simulink model "ComplexPhaseDetectorSwap"  (R2016a)
settings: Solver=VariableStepAuto  StartTime=0.0  StopTime=.05  RelTol=1e-6
PreLoadFcn:
  | Bits = 4
  | Ts=2*3/280e6
  | dBRange=11
  | maxNumErrs=500
  | maxNumBits=1e6
  | AM_Gain=AM_GainDiff;
  | AGC_Gain=AGC_GainCalc;
  | load('IIR_Coeffs.mat');
InitFcn:
  | Br= 1/(10*Ts)
  | FreqOffset=00
  | Mode=2
  | BitsPer=[2,2,1,1]
  | EbNo=50
  | N=6
undefined symbols (not defined in the file or in its folder): designMultirateFIR, DiscIntNeverNeededParam
libraries: xbsIndex_r4 x792, commfilt2 x12, commsink2 x6, dspsigops x4, commrfcorlib x2, commchan3 x2, dspfdesign x2, dspstat3 x2, dspmlti4 x1, commdigbbndpm3 x1, commrandsrc3 x1
(part 1 of 10)
settings Model: Creator=frank.ziegler  LastModifiedBy=frank
settings DebuggingCC: ConsistencyChecking=warning  ArrayBoundsChecking=error  UniqueDataStoreMsg=error

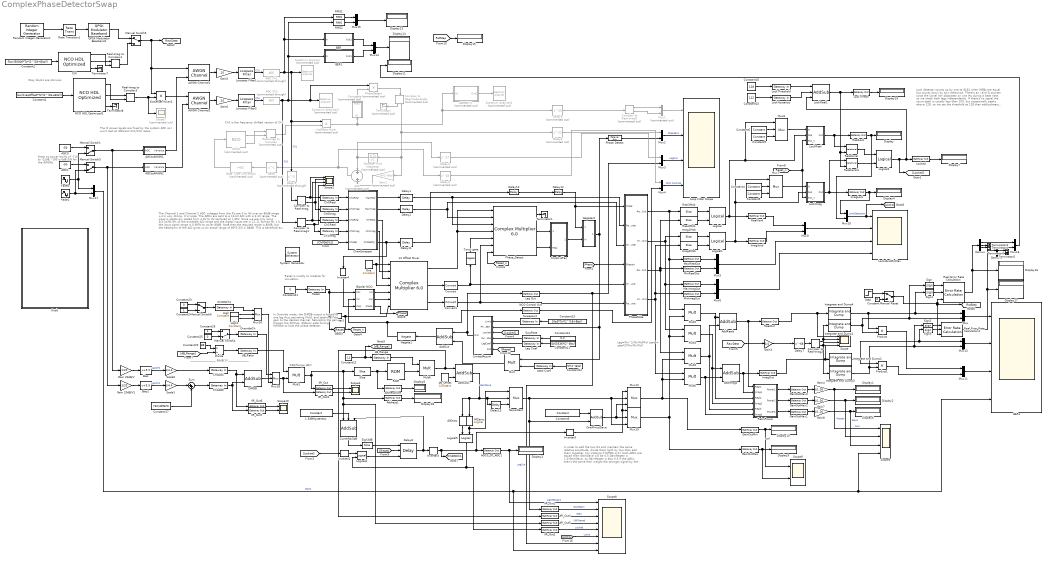
== system ComplexPhaseDetectorSwap ==
  note: Lag=Wn^2/(Kv*Kd*Fs)
      | Lead = zeta*2*Wn/(Kv*Kd)
  note: Lock detector counts up by one to 8191 when MSBs are equal but counts down by two otherwise. There's an I and Q counter since the signal can disappear on one leg during a beat note, so we check both legs independently. If there's no signal the count peak is usually less than 100, but occasionally peaks above 128, so we set the threshold at 128 then add/subtract 112 of hysterisis such that both signals have to drop below 16 to loose lock, then either rise above 240. This gives a strong confidence to the lock and allows the 8192 a long time (76uS) to count down to 256 during a fade.
      | Note, the higher the beat note in the IF, the more false negative at high noise levels. At 800Hz I've seen an error every 10 seconds or so.
  note: Reset is mostly to initialize for simulation
  note: Enter as power levels of -110 to -22dB.
      | -100 is 0dB S/N for the AWGNs
  note: The IF power levels are fixed by the system AGC so I won't test at different Ch1/Ch2 ratios.
  note: Ch2 is the frequency shifted version of Ch1.
  note: The Channel 1 and Channel 2 AGC voltages from the IFs are 0 to 4V over an 80dB range. +4 is very strong, 0 is noise. The AGCs are sent to a 12-bit A/D with a 3.3V range. The input is resistively scaled from 4.0V to 3V centered at 1.65V. Since we are only using 3/3.3=90.9% of the available A/D range and the digital inputs are in 12.11 format for 1.0, the input signal range is 0.909V to cover 80dB.
      | Note that the required range is 80dB, but the headroom of the A/D gives us an actual range of 80*3.3/3 = 88dB. This is beneficial as shown below.
      | We take the difference in AGC voltage between the two channels to define the weighting system based on the stronger signal. If we take the differential and multiply by 8 with saturation this effectively gives us a ± 11dB differential maximum. We can use this to limit the range the combiner attempts to work over since combining is only useful over a 10dB range. The nature of the saturation forces a "Best Source Select" function automatically. We take the sign to define the larger channel. The value addresses a look up table that does the log to linear conversion over a 16384-bit resolution. The Log2Lin transposes the log nature of the AGC to a linear ratio of the two signals. If the two AGCs are the same, the differential is zero and the weights are set to 50-50 for optimal combining. As the difference approaches +1.0, the largest signal gets a weight of 100%.and the other is shut off with a weight of 0%.
  note: In order to add the two IFs and maintain the same relative amplitude, divide them both by two then add them together.
      | For instance if DiffDb is 0 ( both AGCs are equal) then GainSlave will be 0.5.GainMaster = 1.0-GainSlave, so GainMaster is also 0.5
      | If the AGCs aren't the same then weight the stronger signal by the differential.
      | If  GainSlave saturates, ignore the lock and pick the larger signal immediately
  note: In Override mode, the DiffDB output is forced to one leg thus saturating Mult1 and setting all the gain to the desired channel. Saturating the gain triggers the AllOnes, AllZeros gate forcing HardSel to hold the phase detector.
  note: ±88/Range dB/V
  note: ___________________ 88dB/1V _______________
  note: Grey blocks are stimulus
  " System Generator" : xbsIndex_r4/ System Generator  Tag=genX  xilinxfamily=kintex7  part=xc7k325t  speed=-2  package=fbg676  synthesis_tool=Vivado  clock_wrapper=Clock Enables  directory=./netlist  proj_type=Vivado  Synth_file=Vivado Synthesis Defaults  Impl_file=Vivado Implementation Defaults  testbench=off  simulink_period=Ts  sysclk_period=2*3000/280  dcm_input_clock_period=10  incr_netlist=off  trim_vbits=Everywhere in SubSystem  dbl_ovrd=According to Block Masks  core_generation=According to Block Masks  run_coregen=off  deprecated_control=off  eval_field=0  block_type=sysgen
  1.5dBHysteresis : xbsIndex_r4/Constant  const=1.5/11  gui_display_data_type=Fixed-point  arith_type=Signed (2's comp)  n_bits=18  bin_pt=17  preci_type=Single  exp_width=8  frac_width=24  explicit_period=on  period=Ts  equ=P=C  opselect=C  inp2=PCIN>>17  opr=+  inp1=P  carry=CIN  dbl_ovrd=off  block_type=constant
  AD9957-2 : Subsystem  Commented=on
  AGC Ch1 : commrfcorlib/AGC  Commented=through  LegacyMode=off  DetectorMethod=Rectifier  LoopMethod=Linear  UpdatePeriod=100  StepSize=0.1  AdaptationStepSize=0.001  DesiredOutputPower=.05  AveragingLength=100  MaximumGain=30  MaxPowerGain=6  GainOutputPort=off  InputPowerOutputPort=off  SimulateUsing=Interpreted execution
  AGC Ch2 : commrfcorlib/AGC  Commented=through  LegacyMode=off  DetectorMethod=Rectifier  LoopMethod=Linear  UpdatePeriod=100  StepSize=0.1  AdaptationStepSize=0.001  DesiredOutputPower=.05  AveragingLength=100  MaximumGain=30  MaxPowerGain=6  GainOutputPort=off  InputPowerOutputPort=off  SimulateUsing=Interpreted execution
  AGC0 : Constant  Value=-50  OutDataTypeStr=double
  AGC0_GT_AGC1 : xbsIndex_r4/Gateway Out  inherit_from_input=off  hdl_port=on  rows=1  columns=1  UseAsDAC=off  DACChannel='1'  interface=None  automatic_assignment=on  address_offset=hex2dec('00')  intf_name=''  intf_description=''  timing_constraint=None  locs_specified=off  LOCs={}  io_standard={}  block_type=gatewayout
  AGC1 : Constant  Value=-50  OutDataTypeStr=double
  AGCtoAWGN1 : Subsystem
  AGCtoAWGN2 : Subsystem
  AWGN Channel1 : commchan3/AWGN Channel  InputProcessing=Columns as channels (frame based)  seed=67  noiseMode=Variance from port  EbNodB=4  EsNodB=10  SNRdB=10  bitsPerSym=BitsPer(Mode)  Ps=0.707  Tsym=1/Br  variance=1
  AWGN Channel2 : commchan3/AWGN Channel  InputProcessing=Columns as channels (frame based)  seed=70  noiseMode=Variance from port  EbNodB=6  EsNodB=10  SNRdB=10  bitsPerSym=BitsPer(Mode)  Ps=0.707  Tsym=1/Br  variance=1
  Add : Sum  Commented=on  OutDataTypeStr=Inherit: Same as first input
  AddImags : xbsIndex_r4/AddSub  mode=Addition  use_carryin=off  use_carryout=off  en=off  latency=1  precision=User Defined  arith_type="Signed  (2's comp)"  n_bits=18  bin_pt=17  quantization="Round  (unbiased: +/- Inf)"  overflow=Saturate  use_behavioral_HDL=off  hw_selection=Fabric  pipelined=off  dbl_ovrd=off  block_type=addsub
  AddReals : xbsIndex_r4/AddSub  mode=Addition  use_carryin=off  use_carryout=off  en=off  latency=1  precision=User Defined  arith_type="Signed  (2's comp)"  n_bits=18  bin_pt=17  quantization="Round  (unbiased: +/- Inf)"  overflow=Saturate  use_behavioral_HDL=off  hw_selection=Fabric  pipelined=off  dbl_ovrd=off  block_type=addsub
  AddSub : xbsIndex_r4/AddSub  mode=Addition  use_carryin=off  use_carryout=off  en=off  latency=1  precision=User Defined  arith_type="Signed  (2's comp)"  n_bits=18+Bits  bin_pt=0  quantization=Truncate  overflow=Wrap  use_behavioral_HDL=off  hw_selection=Fabric  pipelined=off  dbl_ovrd=off  block_type=addsub
  AddSub1 : xbsIndex_r4/AddSub  mode=Addition  use_carryin=off  use_carryout=off  en=off  latency=1  precision=User Defined  arith_type=Unsigned  n_bits=18  bin_pt=18  quantization=Truncate  overflow=Saturate  use_behavioral_HDL=off  hw_selection=Fabric  pipelined=off  dbl_ovrd=off  block_type=addsub
  Address1 : xbsIndex_r4/Gateway Out  inherit_from_input=off  hdl_port=off  rows=1  columns=1  UseAsDAC=off  DACChannel='1'  interface=None  automatic_assignment=on  address_offset=hex2dec('00')  intf_name=''  intf_description=''  timing_constraint=None  locs_specified=off  LOCs={}  io_standard={}  block_type=gatewayout
  AddressSlice : xbsIndex_r4/Gateway Out  inherit_from_input=off  hdl_port=off  rows=1  columns=1  UseAsDAC=off  DACChannel='1'  interface=None  automatic_assignment=on  address_offset=hex2dec('00')  intf_name=''  intf_description=''  timing_constraint=None  locs_specified=off  LOCs={}  io_standard={}  block_type=gatewayout
  AllOnes : xbsIndex_r4/Logical  logical_function=AND  inputs=1  en=off  latency=0  precision=Full  arith_type=Unsigned  n_bits=16  bin_pt=0  align_bp=on  dbl_ovrd=off  block_type=logical
  AllZeros : xbsIndex_r4/Logical  logical_function=NOR  inputs=1  en=off  latency=0  precision=Full  arith_type=Unsigned  n_bits=16  bin_pt=0  align_bp=on  dbl_ovrd=off  block_type=logical
  BER : Subsystem
  BER1 : Subsystem
  BERs : Scope  NumInputPorts=4
  Bias : Bias  Bias=5.5
  Bias1 : Bias  Bias=5.5
  Bipolar NCO : Subsystem
  CW : dspsigops/NCO HDL Optimized  PhaseIncrementSource=Input port  PhaseIncrement=100  PhaseOffsetSource=Property  PhaseOffset=0  DitherSource=Property  NumDitherBits=4  PhaseQuantization=on  NumQuantizerAccumulatorBits=12  LUTCompress=off  ResetAction=off  ValidInputPort=off  Waveform=Sine and cosine  PhasePort=off  AccumulatorWL=18+Bits  OutputDataType=double  OutputWL=16  OutputFL=14  SimulateUsing=Code generation
  Ch0AGC : xbsIndex_r4/Gateway In  gui_display_data_type=Fixed-point  arith_type=Unsigned  n_bits=13  bin_pt=12  preci_type=Single  exp_width=8  frac_width=24  rows=1  columns=1  quantization="Round  (unbiased: +/- Inf)"  overflow=Saturate  period=Ts  UseAsADC=off  ADCChannel='1'  interface=None  automatic_assignment=on  address_offset=hex2dec('00')  intf_name=''  intf_description=''  default_value=0  timing_constraint=None  locs_specified=off  LOCs={}  io_standard={}  inherit_from_input=off  hdl_port=on  dbl_ovrd=off  block_type=gatewayin
  Ch0GtCh1 : xbsIndex_r4/Gateway In  gui_display_data_type=Boolean  arith_type=Boolean  n_bits=18  bin_pt=9  preci_type=Single  exp_width=8  frac_width=24  rows=1  columns=1  quantization="Round  (unbiased: +/- Inf)"  overflow=Wrap  period=Ts  UseAsADC=off  ADCChannel='1'  interface=None  automatic_assignment=on  address_offset=hex2dec('00')  intf_name='axi4'  intf_description='Lead Coefficient'  default_value=10  timing_constraint=None  locs_specified=off  LOCs={}  io_standard={}  inherit_from_input=off  hdl_port=on  dbl_ovrd=off  block_type=gatewayin
  Ch0Imag : xbsIndex_r4/Gateway In  gui_display_data_type=Fixed-point  arith_type="Signed  (2's comp)"  n_bits=18  bin_pt=17  preci_type=Single  exp_width=8  frac_width=24  rows=1  columns=1  quantization="Round  (unbiased: +/- Inf)"  overflow=Saturate  period=Ts  UseAsADC=off  ADCChannel='1'  interface=None  automatic_assignment=on  address_offset=hex2dec('00')  intf_name=''  intf_description=''  default_value=0  timing_constraint=None  locs_specified=off  LOCs={}  io_standard={}  inherit_from_input=off  hdl_port=on  dbl_ovrd=off  block_type=gatewayin
  Ch0Real : xbsIndex_r4/Gateway In  gui_display_data_type=Fixed-point  arith_type="Signed  (2's comp)"  n_bits=18  bin_pt=17  preci_type=Single  exp_width=8  frac_width=24  rows=1  columns=1  quantization="Round  (unbiased: +/- Inf)"  overflow=Saturate  period=Ts  UseAsADC=off  ADCChannel='1'  interface=None  automatic_assignment=on  address_offset=hex2dec('00')  intf_name=''  intf_description=''  default_value=0  timing_constraint=None  locs_specified=off  LOCs={}  io_standard={}  inherit_from_input=off  hdl_port=on  dbl_ovrd=off  block_type=gatewayin
  Ch1AGC : xbsIndex_r4/Gateway In  gui_display_data_type=Fixed-point  arith_type=Unsigned  n_bits=13  bin_pt=12  preci_type=Single  exp_width=8  frac_width=24  rows=1  columns=1  quantization="Round  (unbiased: +/- Inf)"  overflow=Saturate  period=Ts  UseAsADC=off  ADCChannel='1'  interface=None  automatic_assignment=on  address_offset=hex2dec('00')  intf_name=''  intf_description=''  default_value=0  timing_constraint=None  locs_specified=off  LOCs={}  io_standard={}  inherit_from_input=off  hdl_port=on  dbl_ovrd=off  block_type=gatewayin
  Ch1Imag : xbsIndex_r4/Gateway In  gui_display_data_type=Fixed-point  arith_type="Signed  (2's comp)"  n_bits=18  bin_pt=17  preci_type=Single  exp_width=8  frac_width=24  rows=1  columns=1  quantization="Round  (unbiased: +/- Inf)"  overflow=Saturate  period=Ts  UseAsADC=off  ADCChannel='1'  interface=None  automatic_assignment=on  address_offset=hex2dec('00')  intf_name=''  intf_description=''  default_value=0  timing_constraint=None  locs_specified=off  LOCs={}  io_standard={}  inherit_from_input=off  hdl_port=on  dbl_ovrd=off  block_type=gatewayin
  Ch1Real : xbsIndex_r4/Gateway In  gui_display_data_type=Fixed-point  arith_type="Signed  (2's comp)"  n_bits=18  bin_pt=17  preci_type=Single  exp_width=8  frac_width=24  rows=1  columns=1  quantization="Round  (unbiased: +/- Inf)"  overflow=Saturate  period=Ts  UseAsADC=off  ADCChannel='1'  interface=None  automatic_assignment=on  address_offset=hex2dec('00')  intf_name=''  intf_description=''  default_value=0  timing_constraint=None  locs_specified=off  LOCs={}  io_standard={}  inherit_from_input=off  hdl_port=on  dbl_ovrd=off  block_type=gatewayin
  ChanSwapper : Subsystem
  Complex to Magnitude-Angle : ComplexToMagnitudeAngle  Commented=on
  Complex to Real-Imag : ComplexToRealImag
  Complex to Real-Imag1 : ComplexToRealImag
  Complex to Real-Imag2 : ComplexToRealImag
  Complex to Real-Imag5 : ComplexToRealImag  Commented=on
  Conju gate : xbsIndex_r4/Negate  precision=User Defined  arith_type="Signed  (2's comp)"  n_bits=18  bin_pt=17  quantization=Truncate  overflow=Saturate  en=off  latency=0  dbl_ovrd=off  block_type=negate
  Conjugate : Subsystem  Commented=on
  Constant : Constant  Value=0
  Constant1 : Constant  Value=floor(FreqOffset*Ts*(2^(18+Bits)))  OutDataTypeStr=int32  SampleTime=Ts
  Constant10 : Constant  Value=128
  Constant11 : Constant  Value=50/65536*(2^Bits)  OutDataTypeStr=double
  Constant12 : Constant  Value=5*(2^Bits)  OutDataTypeStr=double
  Constant13 : Constant  Value=10e3*Ts*(2^(18+Bits))  OutDataTypeStr=double
  Constant14 : Constant  Value=0.2  OutDataTypeStr=double
  Constant15 : Constant  Value=112
  Constant17 : Constant  Value=732/4096*0
  Constant2 : Constant  Value=floor(50000*Ts*(2^(18+Bits)))  OutDataTypeStr=int32  SampleTime=Ts
  Constant20 : Constant  Value=88  OutDataTypeStr=double
  Constant21 : Constant  Value=0  OutDataTypeStr=double
  Constant22 : Constant  Value=11  OutDataTypeStr=double
  Constant23 : Constant  Value=0  OutDataTypeStr=double
  Constant24 : Constant  OutDataTypeStr=double
  Constant25 : Constant  Value=0  OutDataTypeStr=double
  Constant26 : Constant  OutDataTypeStr=double
  Constant3 : xbsIndex_r4/Constant  const=1.0  gui_display_data_type=Fixed-point  arith_type=Unsigned  n_bits=18  bin_pt=18  preci_type=Single  exp_width=8  frac_width=24  explicit_period=on  period=Ts  equ=P=C  opselect=C  inp2=PCIN>>17  opr=+  inp1=P  carry=CIN  dbl_ovrd=off  block_type=constant
  Constant4 : xbsIndex_r4/Constant  const=1  gui_display_data_type=Fixed-point  arith_type=Unsigned  n_bits=8  bin_pt=0  preci_type=Single  exp_width=8  frac_width=24  explicit_period=off  period=1  equ=P=C  opselect=C  inp2=PCIN>>17  opr=+  inp1=P  carry=CIN  dbl_ovrd=off  block_type=constant
  Constant5 : xbsIndex_r4/Constant  const=2  gui_display_data_type=Fixed-point  arith_type=Unsigned  n_bits=8  bin_pt=0  preci_type=Single  exp_width=8  frac_width=24  explicit_period=off  period=1  equ=P=C  opselect=C  inp2=PCIN>>17  opr=+  inp1=P  carry=CIN  dbl_ovrd=off  block_type=constant
  Constant6 : xbsIndex_r4/Constant  const=1  gui_display_data_type=Fixed-point  arith_type=Unsigned  n_bits=8  bin_pt=0  preci_type=Single  exp_width=8  frac_width=24  explicit_period=off  period=1  equ=P=C  opselect=C  inp2=PCIN>>17  opr=+  inp1=P  carry=CIN  dbl_ovrd=off  block_type=constant
  Constant9 : xbsIndex_r4/Constant  const=2  gui_display_data_type=Fixed-point  arith_type=Unsigned  n_bits=8  bin_pt=0  preci_type=Single  exp_width=8  frac_width=24  explicit_period=off  period=1  equ=P=C  opselect=C  inp2=PCIN>>17  opr=+  inp1=P  carry=CIN  dbl_ovrd=off  block_type=constant
  Convert : xbsIndex_r4/Convert  gui_display_data_type=Fixed-point  arith_type="Signed  (2's comp)"  n_bits=18  bin_pt=17  float_type=Single  exp_bits=8  fraction_bits=24  quantization=Truncate  overflow=Saturate  en=off  latency=1  pipeline=off  dbl_ovrd=off  block_type=convert
  Convert1 : xbsIndex_r4/Convert  gui_display_data_type=Fixed-point  arith_type="Signed  (2's comp)"  n_bits=18  bin_pt=17  float_type=Single  exp_bits=8  fraction_bits=24  quantization=Truncate  overflow=Saturate  en=off  latency=1  pipeline=off  dbl_ovrd=off  block_type=convert
  Cordic ATan : Subsystem
  Current±3dB : xbsIndex_r4/AddSub  mode=Addition or Subtraction  use_carryin=off  use_carryout=off  en=off  latency=0  precision=User Defined  arith_type="Signed  (2's comp)"  n_bits=12  bin_pt=11  quantization=Truncate  overflow=Saturate  use_behavioral_HDL=off  hw_selection=Fabric  pipelined=off  dbl_ovrd=off  block_type=addsub
  Data Type Conversion : DataTypeConversion  Commented=on  OutDataTypeStr=int32  SaturateOnIntegerOverflow=on
  Delay : Delay  Commented=on  DelayLength=1
  Delay1 : xbsIndex_r4/Delay  rst=off  infoeditControl=Selection of Reset will increase slice count due to use of real FFs and instead of SRLs  en=off  latency=4  reg_retiming=off  dbl_ovrd=off  block_type=delay
  Delay10 : xbsIndex_r4/Delay  rst=off  infoeditControl=Selection of Reset will increase slice count due to use of real FFs and instead of SRLs  en=off  latency=3  reg_retiming=off  dbl_ovrd=off  block_type=delay
  Delay11 : xbsIndex_r4/Delay  rst=off  infoeditControl=Selection of Reset will increase slice count due to use of real FFs and instead of SRLs  en=off  latency=4  reg_retiming=off  dbl_ovrd=off  block_type=delay
  Delay12 : xbsIndex_r4/Delay  rst=off  infoeditControl=Selection of Reset will increase slice count due to use of real FFs and instead of SRLs  en=off  latency=17  reg_retiming=off  dbl_ovrd=off  block_type=delay
  Delay13 : xbsIndex_r4/Delay  rst=off  infoeditControl=Selection of Reset will increase slice count due to use of real FFs and instead of SRLs  en=off  latency=1  reg_retiming=off  dbl_ovrd=off  block_type=delay
  Delay2 : xbsIndex_r4/Delay  rst=off  infoeditControl=Selection of Reset will increase slice count due to use of real FFs and instead of SRLs  en=off  latency=4  reg_retiming=off  dbl_ovrd=off  block_type=delay
  Delay3 : Delay  Commented=on  DelayLength=27
  Delay4 : Delay  Commented=on  DelayLength=28
  Delay5 : Delay  Commented=on  DelayLength=23
  Delay6 : Delay  Commented=on  DelayLength=23
  Delay7 : Delay  DelayLength=68
  Delay8 : xbsIndex_r4/Delay  rst=on  infoeditControl=Selection of Reset will increase slice count due to use of real FFs and instead of SRLs  en=on  latency=1  reg_retiming=off  dbl_ovrd=off  block_type=delay
  Delay9 : Delay  Commented=through  DelayLength=3
  Demux : Demux  Outputs=3
  Demux1 : Demux  Outputs=3
  DiffDB : xbsIndex_r4/AddSub  mode=Subtraction  use_carryin=off  use_carryout=off  en=off  latency=1  precision=Full  arith_type="Signed  (2's comp)"  n_bits=13  bin_pt=12  quantization=Truncate  overflow=Saturate  use_behavioral_HDL=off  hw_selection=Fabric  pipelined=off  dbl_ovrd=off  block_type=addsub
  Discrete-Time Integrator : DiscreteIntegrator  Commented=on  gainval=(2^Bits)*50/65536/Ts  InitialConditionSetting=State (most efficient)  SampleTime=Ts  ICPrevOutput=DiscIntNeverNeededParam  ICPrevScaledInput=DiscIntNeverNeededParam
  Display{,1..4,6..11,13..19} (18 alike) : Display
      Display11 settings: Format=short_e
      Display14 settings: Format=short_e
  Divide : Product  Inputs=*/
  ExtOffset Mixer1 : Product
  Fade0 : Sin  Amplitude=10  Bias=-90  Frequency=5000*pi()  SampleTime=Ts
  Fade1 : Sin  Amplitude=10  Bias=-90  Frequency=5000*pi()  Phase=pi()  SampleTime=Ts
  Gain 20dB/V : Gain  Gain=1/20
  Gain 20dB/V1 : Gain  Gain=1/20
  Gain1 : Gain  Commented=on  Gain=5*(2^Bits)
  Gain3 : Gain  Gain=1/4
  Gain4 : Gain  Gain=1/1.26
  Gain5 : Gain  Gain=.25
  Gain6 : Gain  Gain=.25
  Gain7 : Gain  Gain=1/1.26
  Gain8 : Gain  Gain=1/1.26
  GainOutMax : xbsIndex_r4/Gateway Out  inherit_from_input=off  hdl_port=on  rows=1  columns=1  UseAsDAC=off  DACChannel='1'  interface=None  automatic_assignment=on  address_offset=hex2dec('00')  intf_name=''  intf_description=''  timing_constraint=None  locs_specified=off  LOCs={}  io_standard={}  block_type=gatewayout
  GainOutMax1 : xbsIndex_r4/Gateway Out  inherit_from_input=off  hdl_port=off  rows=1  columns=1  UseAsDAC=off  DACChannel='1'  interface=None  automatic_assignment=on  address_offset=hex2dec('00')  intf_name=''  intf_description=''  timing_constraint=None  locs_specified=off  LOCs={}  io_standard={}  block_type=gatewayout
  GainOutMax2 : xbsIndex_r4/Gateway Out  inherit_from_input=off  hdl_port=off  rows=1  columns=1  UseAsDAC=off  DACChannel='1'  interface=None  automatic_assignment=on  address_offset=hex2dec('00')  intf_name=''  intf_description=''  timing_constraint=None  locs_specified=off  LOCs={}  io_standard={}  block_type=gatewayout
  GainOutMax3 : xbsIndex_r4/Gateway Out  inherit_from_input=off  hdl_port=off  rows=1  columns=1  UseAsDAC=off  DACChannel='1'  interface=None  automatic_assignment=on  address_offset=hex2dec('00')  intf_name=''  intf_description=''  timing_constraint=None  locs_specified=off  LOCs={}  io_standard={}  block_type=gatewayout
  GainOutMin : xbsIndex_r4/Gateway Out  inherit_from_input=off  hdl_port=on  rows=1  columns=1  UseAsDAC=off  DACChannel='1'  interface=None  automatic_assignment=on  address_offset=hex2dec('00')  intf_name=''  intf_description=''  timing_constraint=None  locs_specified=off  LOCs={}  io_standard={}  block_type=gatewayout
  High : xbsIndex_r4/Constant  const=.75  gui_display_data_type=Fixed-point  arith_type=Signed (2's comp)  n_bits=14  bin_pt=12  preci_type=Single  exp_width=8  frac_width=24  explicit_period=on  period=Ts  equ=P=C  opselect=C  inp2=PCIN>>17  opr=+  inp1=P  carry=CIN  dbl_ovrd=off  block_type=constant
  High1 : xbsIndex_r4/Constant  const=-.75  gui_display_data_type=Fixed-point  arith_type=Signed (2's comp)  n_bits=14  bin_pt=12  preci_type=Single  exp_width=8  frac_width=24  explicit_period=on  period=Ts  equ=P=C  opselect=C  inp2=PCIN>>17  opr=+  inp1=P  carry=CIN  dbl_ovrd=off  block_type=constant
  IIR_Out{,1..7} (8 alike) : xbsIndex_r4/Gateway Out  inherit_from_input=off  hdl_port=off  rows=1  columns=1  UseAsDAC=off  DACChannel='1'  interface=None  automatic_assignment=on  address_offset=hex2dec('00')  intf_name=''  intf_description=''  timing_constraint=None  locs_specified=off  LOCs={}  io_standard={}  block_type=gatewayout
  Imag1Msb : xbsIndex_r4/Slice  nbits=1  boolean_output=on  mode=Upper Bit Location + Width  bit1=0  base1=MSB of Input  bit0=0  base0=LSB of Input  dbl_ovrd=off  block_type=slice
  Imag2Msb : xbsIndex_r4/Slice  nbits=1  boolean_output=on  mode=Upper Bit Location + Width  bit1=0  base1=MSB of Input  bit0=0  base0=LSB of Input  dbl_ovrd=off  block_type=slice
  ImagLock : xbsIndex_r4/Gateway Out  inherit_from_input=off  hdl_port=on  rows=1  columns=1  UseAsDAC=off  DACChannel='1'  interface=None  automatic_assignment=on  address_offset=hex2dec('00')  intf_name=''  intf_description=''  timing_constraint=None  locs_specified=off  LOCs={}  io_standard={}  block_type=gatewayout
  ImagOut : xbsIndex_r4/Gateway Out  inherit_from_input=off  hdl_port=on  rows=1  columns=1  UseAsDAC=off  DACChannel='1'  interface=None  automatic_assignment=on  address_offset=hex2dec('00')  intf_name=''  intf_description=''  timing_constraint=None  locs_specified=off  LOCs={}  io_standard={}  block_type=gatewayout
  ImagXord : xbsIndex_r4/Gateway Out  inherit_from_input=off  hdl_port=on  rows=1  columns=1  UseAsDAC=off  DACChannel='1'  interface=None  automatic_assignment=on  address_offset=hex2dec('00')  intf_name=''  intf_description=''  timing_constraint=None  locs_specified=off  LOCs={}  io_standard={}  block_type=gatewayout
  Int Offset Mixer : xbsIndex_r4/Complex Multiplier 6.0   hasatlast=off  hasatuser=off  atuserwidth=1  hasbtlast=off  hasbtuser=off  btuserwidth=1  multtype=Use_Mults  optimizegoal=Resources  flowcontrol=NonBlocking  outputwidth=20  roundmode=Truncate  hasctrltlast=off  hasctrltuser=off  ctrltuserwidth=1  outtlastbehv=Null  latencyconfig=Manual  minimumlatency=3  aclken=off  aresetn=on  trim_axipin_name=on  simulation_type=hybrid_sim  simulation_model=sysgen:cmpy_v6_0  data_path_portlist={ 's_axis_a_tdata_real', 's_axis_a_tdata_imag', 's_axis_b_tdata_real', 's_axis_b_tdata_imag', 's_axis_ctrl_tdata_rounding_bit', 'm_axis_dout_tdata_real', 'm_axis_dout_tdata_imag' }  aportwidth=63  bportwidth=63  ip_name=Complex Multiplier  ip_version=6.0  dsptool_ready=true  ipcore_usecache=true  ipcore_useipmodelcache=true  ipcore_verbose=false  ipcore_latency_parameter='minimumlatency'  wrapper_available=true  port_translation_map={ 'aclken' => 'en', 'aresetn' => 'rst'}  block_type=cmpy_v6_0
  IntOffset Mixer : Product  Commented=on
  Integrate and Dump{1..4} (4 alike) : commfilt2/Integrate and Dump  obssamples=1/(Br*Ts)  offsetsamples=8  nodump=off  roundingMode=Floor  overflowMode=off  outputDataTypeStr=Inherit: Same as accumulator  outputLastDataTypeStr=Inherit: Same as accumulator
  Inverter{1..5} (5 alike) : xbsIndex_r4/Inverter  en=off  latency=0  dbl_ovrd=off  block_type=inv
  Knob : Subsystem  DialogController=hmiCreateDDGDialog  IsWebBlock=on  mask(MWDashboardBlock){webBlockId=e460d0c1-8f1d-4963-a065-60dc3f9fc9ee, webBlockType=continuousknob, ShowInLibBrowser=on, ShowInitialText=on, HMISrcModelName=ComplexPhaseDetectorSwap}
      mask prompts: webBlockId "WebBlock Id"; webBlockType "WebBlock Type"; HMISrcModelName "Source Model"
      mask Help: helpview([docroot '/mapfiles/simulink.map'], 'hmi_knob')
      mask Display:
      | if strcmp(get_param(bdroot(gcb),'BlockDiagramType'), 'library')
      |     image([(matlabroot) '/toolbox/simulink/hmi/icons/ContinuousKnob.png']);
      | end
  Lag Coef : xbsIndex_r4/Gateway In  gui_display_data_type=Fixed-point  arith_type=Unsigned  n_bits=18  bin_pt=17  preci_type=Single  exp_width=8  frac_width=24  rows=1  columns=1  quantization="Round  (unbiased: +/- Inf)"  overflow=Wrap  period=Ts  UseAsADC=off  ADCChannel='1'  interface=None  automatic_assignment=on  address_offset=hex2dec('00')  intf_name='axi4'  intf_description='Lead Coefficient'  default_value=5*Ts  timing_constraint=None  locs_specified=off  LOCs={}  io_standard={}  inherit_from_input=off  hdl_port=on  dbl_ovrd=off  block_type=gatewayin
  Lag Out : xbsIndex_r4/Gateway Out  inherit_from_input=off  hdl_port=on  rows=1  columns=1  UseAsDAC=off  DACChannel='1'  interface=None  automatic_assignment=on  address_offset=hex2dec('00')  intf_name=''  intf_description=''  timing_constraint=None  locs_specified=off  LOCs={}  io_standard={}  block_type=gatewayout
  Lead Coef : xbsIndex_r4/Gateway In  gui_display_data_type=Fixed-point  arith_type=Unsigned  n_bits=18  bin_pt=9  preci_type=Single  exp_width=8  frac_width=24  rows=1  columns=1  quantization="Round  (unbiased: +/- Inf)"  overflow=Wrap  period=Ts  UseAsADC=off  ADCChannel='1'  interface=None  automatic_assignment=on  address_offset=hex2dec('00')  intf_name='axi4'  intf_description='Lead Coefficient'  default_value=10  timing_constraint=None  locs_specified=off  LOCs={}  io_standard={}  inherit_from_input=off  hdl_port=on  dbl_ovrd=off  block_type=gatewayin
  LimitedAccum : Subsystem
  LockHysterisis : xbsIndex_r4/Gateway In  gui_display_data_type=Fixed-point  arith_type=Unsigned  n_bits=13  bin_pt=0  preci_type=Single  exp_width=8  frac_width=24  rows=1  columns=1  quantization="Round  (unbiased: +/- Inf)"  overflow=Wrap  period=Ts  UseAsADC=off  ADCChannel='1'  interface=None  automatic_assignment=on  address_offset=hex2dec('00')  intf_name=''  intf_description=''  default_value=0  timing_constraint=None  locs_specified=off  LOCs={}  io_standard={}  inherit_from_input=off  hdl_port=on  dbl_ovrd=off  block_type=gatewayin
  LockImag : Subsystem
  LockReal : Subsystem
  LockReal1 : xbsIndex_r4/AddSub  mode=Addition or Subtraction  use_carryin=off  use_carryout=off  en=off  latency=0  precision=User Defined  arith_type=Unsigned  n_bits=13  bin_pt=0  quantization=Truncate  overflow=Wrap  use_behavioral_HDL=off  hw_selection=Fabric  pipelined=off  dbl_ovrd=off  block_type=addsub
  LockThresh : xbsIndex_r4/Gateway Out  inherit_from_input=off  hdl_port=off  rows=1  columns=1  UseAsDAC=off  DACChannel='1'  interface=None  automatic_assignment=on  address_offset=hex2dec('00')  intf_name=''  intf_description=''  timing_constraint=None  locs_specified=off  LOCs={}  io_standard={}  block_type=gatewayout
  LockThreshold : xbsIndex_r4/Gateway In  gui_display_data_type=Fixed-point  arith_type=Unsigned  n_bits=13  bin_pt=0  preci_type=Single  exp_width=8  frac_width=24  rows=1  columns=1  quantization="Round  (unbiased: +/- Inf)"  overflow=Wrap  period=Ts  UseAsADC=off  ADCChannel='1'  interface=None  automatic_assignment=on  address_offset=hex2dec('00')  intf_name=''  intf_description=''  default_value=0  timing_constraint=None  locs_specified=off  LOCs={}  io_standard={}  inherit_from_input=off  hdl_port=on  dbl_ovrd=off  block_type=gatewayin
  Locked : xbsIndex_r4/Gateway Out  inherit_from_input=off  hdl_port=on  rows=1  columns=1  UseAsDAC=off  DACChannel='1'  interface=None  automatic_assignment=on  address_offset=hex2dec('00')  intf_name=''  intf_description=''  timing_constraint=None  locs_specified=off  LOCs={}  io_standard={}  block_type=gatewayout
  LocksAndMinMax : Scope  NumInputPorts=4
  Logical : xbsIndex_r4/Logical  logical_function=XOR  inputs=2  en=off  latency=1  precision=Full  arith_type=Unsigned  n_bits=16  bin_pt=0  align_bp=on  dbl_ovrd=off  block_type=logical
  Logical1 : xbsIndex_r4/Logical  logical_function=XOR  inputs=2  en=off  latency=1  precision=Full  arith_type=Unsigned  n_bits=16  bin_pt=0  align_bp=on  dbl_ovrd=off  block_type=logical
  Logical2 : xbsIndex_r4/Logical  logical_function=OR  inputs=2  en=off  latency=1  precision=Full  arith_type=Boolean  n_bits=16  bin_pt=0  align_bp=on  dbl_ovrd=off  block_type=logical
  Logical4 : xbsIndex_r4/Logical  logical_function=OR  inputs=2  en=off  latency=0  precision=Full  arith_type=Unsigned  n_bits=16  bin_pt=0  align_bp=on  dbl_ovrd=off  block_type=logical
  Logical5 : xbsIndex_r4/Logical  logical_function=OR  inputs=2  en=off  latency=0  precision=Full  arith_type=Unsigned  n_bits=16  bin_pt=0  align_bp=on  dbl_ovrd=off  block_type=logical
  Loop Filter Scope : Scope  NumInputPorts=4
  Lowpass Filter1 : dspfdesign/Lowpass Filter  FilterType=FIR  DesignForMinimumOrder=off  FilterOrder=26  PassbandFrequency=Br/2  StopbandFrequency=Br*2  PassbandRipple=0.1  StopbandAttenuation=80  InheritSampleRate=off  SampleRate=1/Ts  roundingMode=Floor  coeffsDataTypeStr=fixdt(1,16)  SimulateUsing=Interpreted execution
  Lowpass Filter2 : dspfdesign/Lowpass Filter  FilterType=FIR  DesignForMinimumOrder=off  FilterOrder=26  PassbandFrequency=Br/2  StopbandFrequency=Br*2  PassbandRipple=0.1  StopbandAttenuation=80  InheritSampleRate=off  SampleRate=1/Ts  roundingMode=Floor  coeffsDataTypeStr=fixdt(1,16)  SimulateUsing=Interpreted execution
  Manual Reset : ManualSwitch
  Manual Switch1 : ManualSwitch  CurrentSetting=0
  Manual Switch3 : ManualSwitch  CurrentSetting=0
  Manual Switch4 : ManualSwitch  CurrentSetting=0
  Manual Switch5 : ManualSwitch
  Manual Switch6 : ManualSwitch
  MaxImagOut : xbsIndex_r4/Gateway Out  inherit_from_input=off  hdl_port=on  rows=1  columns=1  UseAsDAC=off  DACChannel='1'  interface=None  automatic_assignment=on  address_offset=hex2dec('00')  intf_name=''  intf_description=''  timing_constraint=None  locs_specified=off  LOCs={}  io_standard={}  block_type=gatewayout
  MaxRealOut : xbsIndex_r4/Gateway Out  inherit_from_input=off  hdl_port=on  rows=1  columns=1  UseAsDAC=off  DACChannel='1'  interface=None  automatic_assignment=on  address_offset=hex2dec('00')  intf_name=''  intf_description=''  timing_constraint=None  locs_specified=off  LOCs={}  io_standard={}  block_type=gatewayout
  MinImagOut : xbsIndex_r4/Gateway Out  inherit_from_input=off  hdl_port=on  rows=1  columns=1  UseAsDAC=off  DACChannel='1'  interface=None  automatic_assignment=on  address_offset=hex2dec('00')  intf_name=''  intf_description=''  timing_constraint=None  locs_specified=off  LOCs={}  io_standard={}  block_type=gatewayout
  MinRealOut : xbsIndex_r4/Gateway Out  inherit_from_input=off  hdl_port=on  rows=1  columns=1  UseAsDAC=off  DACChannel='1'  interface=None  automatic_assignment=on  address_offset=hex2dec('00')  intf_name=''  intf_description=''  timing_constraint=None  locs_specified=off  LOCs={}  io_standard={}  block_type=gatewayout
  Mult : xbsIndex_r4/Mult  precision=User Defined  arith_type="Signed  (2's comp)"  n_bits=18+Bits  bin_pt=9  quantization="Round  (unbiased: +/- Inf)"  overflow=Wrap  en=off  latency=4  use_behavioral_HDL=off  opt=Speed  use_embedded=on  optimum_pipeline=off  pipeline=on  dbl_ovrd=off  use_rpm=on  placement_style=Triangular  block_type=mult
  Mult1 : xbsIndex_r4/Mult  precision=User Defined  arith_type="Signed  (2's comp)"  n_bits=18  bin_pt=17  quantization=Truncate  overflow=Saturate  en=off  latency=3  use_behavioral_HDL=off  opt=Speed  use_embedded=on  optimum_pipeline=off  pipeline=on  dbl_ovrd=off  use_rpm=on  placement_style=Triangular  block_type=mult
  Mult{2..5} (4 alike) : xbsIndex_r4/Mult  precision=User Defined  arith_type="Signed  (2's comp)"  n_bits=18  bin_pt=17  quantization="Round  (unbiased: +/- Inf)"  overflow=Flag as error  en=off  latency=3  use_behavioral_HDL=off  opt=Speed  use_embedded=on  optimum_pipeline=off  pipeline=on  dbl_ovrd=off  use_rpm=on  placement_style=Triangular  block_type=mult
  Mult6 : xbsIndex_r4/Mult  precision=User Defined  arith_type="Signed  (2's comp)"  n_bits=18  bin_pt=17  quantization=Truncate  overflow=Saturate  en=off  latency=3  use_behavioral_HDL=off  opt=Speed  use_embedded=on  optimum_pipeline=off  pipeline=on  dbl_ovrd=off  use_rpm=on  placement_style=Triangular  block_type=mult
  Mux{,2..6,9..11,13..17} (14 alike) : Mux  Inputs=2
  Mux1 : Mux  Commented=on  Inputs=2
  Mux{7..8,12,18..20} (6 alike) : xbsIndex_r4/Mux  inputs=2  en=off  latency=0  precision=Full  arith_type=Unsigned  n_bits=16  bin_pt=14  quantization=Truncate  overflow=Wrap  dbl_ovrd=off  block_type=mux
  NCO HDL Optimized1 : dspsigops/NCO HDL Optimized  PhaseIncrementSource=Input port  PhaseIncrement=100  PhaseOffsetSource=Property  PhaseOffset=0*2^(18+Bits)/8  DitherSource=Property  NumDitherBits=4  PhaseQuantization=on  NumQuantizerAccumulatorBits=12  LUTCompress=off  ResetAction=off  ValidInputPort=off  Waveform=Sine and cosine  PhasePort=off  AccumulatorWL=18+Bits  OutputDataType=double  OutputWL=16  OutputFL=14  SimulateUsing=Code generation
  NCO Control Out : xbsIndex_r4/Gateway Out  inherit_from_input=off  hdl_port=on  rows=1  columns=1  UseAsDAC=off  DACChannel='1'  interface=None  automatic_assignment=on  address_offset=hex2dec('00')  intf_name=''  intf_description=''  timing_constraint=None  locs_specified=off  LOCs={}  io_standard={}  block_type=gatewayout
  NCO1 : dspsigops/NCO  Commented=on  AccIncSrc=Input port  AccInc=100  PhaseOffsetSrc=Specify via dialog  PhaseOffset=0  AccumWL=18+Bits  HasDither=off  DitherWL=4  PNgeneratorLength=19  HasPhaseQuantizer=off  TableDepth=12  HasOutputPhaseError=off  Formula=Sine and cosine  DataType=double  OutputWL=16  OutputFL=14  CompMethod=Table lookup (no interpolation)  SampleTime=Ts  SamplesPerFrame=1  OutputFrames=off
  Negate1 : xbsIndex_r4/Negate  precision=User Defined  arith_type="Signed  (2's comp)"  n_bits=18+Bits  bin_pt=0  quantization=Truncate  overflow=Saturate  en=off  latency=1  dbl_ovrd=off  block_type=negate
  Negater2 : Subsystem
  NeverZero : xbsIndex_r4/Mux  inputs=2  en=off  latency=0  precision=Full  arith_type=Unsigned  n_bits=16  bin_pt=14  quantization=Truncate  overflow=Wrap  dbl_ovrd=off  block_type=mux
  One : xbsIndex_r4/Constant  const=1  gui_display_data_type=Boolean  arith_type=Boolean  n_bits=18  bin_pt=17  preci_type=Single  exp_width=8  frac_width=24  explicit_period=on  period=Ts  equ=P=C  opselect=C  inp2=PCIN>>17  opr=+  inp1=P  carry=CIN  dbl_ovrd=off  block_type=constant
  OneMinusSlave : xbsIndex_r4/AddSub  mode=Subtraction  use_carryin=off  use_carryout=off  en=off  latency=0  precision=User Defined  arith_type=Unsigned  n_bits=18  bin_pt=18  quantization=Truncate  overflow=Wrap  use_behavioral_HDL=off  hw_selection=Fabric  pipelined=off  dbl_ovrd=off  block_type=addsub
  OverrideCh : xbsIndex_r4/Gateway In  gui_display_data_type=Boolean  arith_type=Boolean  n_bits=18  bin_pt=9  preci_type=Single  exp_width=8  frac_width=24  rows=1  columns=1  quantization="Round  (unbiased: +/- Inf)"  overflow=Wrap  period=Ts  UseAsADC=off  ADCChannel='1'  interface=None  automatic_assignment=on  address_offset=hex2dec('00')  intf_name='axi4'  intf_description='Lead Coefficient'  default_value=10  timing_constraint=None  locs_specified=off  LOCs={}  io_standard={}  inherit_from_input=off  hdl_port=on  dbl_ovrd=off  block_type=gatewayin
  Phase Detect : xbsIndex_r4/Gateway Out  inherit_from_input=off  hdl_port=on  rows=1  columns=1  UseAsDAC=off  DACChannel='1'  interface=None  automatic_assignment=on  address_offset=hex2dec('00')  intf_name=''  intf_description=''  timing_constraint=None  locs_specified=off  LOCs={}  io_standard={}  block_type=gatewayout
  PhaseDetect : Product  Commented=on
  PhaseSlide : Subsystem
  Phase_Detect : xbsIndex_r4/Complex Multiplier 6.0   hasatlast=off  hasatuser=off  atuserwidth=1  hasbtlast=off  hasbtuser=off  btuserwidth=1  multtype=Use_Mults  optimizegoal=Resources  flowcontrol=NonBlocking  outputwidth=18  roundmode=Truncate  hasctrltlast=off  hasctrltuser=off  ctrltuserwidth=1  outtlastbehv=Null  latencyconfig=Automatic  minimumlatency=37  aclken=off  aresetn=on  trim_axipin_name=on  simulation_type=hybrid_sim  simulation_model=sysgen:cmpy_v6_0  data_path_portlist={ 's_axis_a_tdata_real', 's_axis_a_tdata_imag', 's_axis_b_tdata_real', 's_axis_b_tdata_imag', 's_axis_ctrl_tdata_rounding_bit', 'm_axis_dout_tdata_real', 'm_axis_dout_tdata_imag' }  aportwidth=63  bportwidth=63  ip_name=Complex Multiplier  ip_version=6.0  dsptool_ready=true  ipcore_usecache=true  ipcore_useipmodelcache=true  ipcore_verbose=false  ipcore_latency_parameter='minimumlatency'  wrapper_available=true  port_translation_map={ 'aclken' => 'en', 'aresetn' => 'rst'}  block_type=cmpy_v6_0
  Product : Product
  Product1 : Product
  QPSK Modulator Baseband1 : commdigbbndpm3/QPSK Modulator Baseband  InType=Integer  Enc=Gray  Ph=pi/4  outDtype=double  outWordLen=16  outUDDataType=sfix(16)  outFracLenMode=Best precision  outFracLen=15  outDataTypeStr=double  outLastDataTypeStr=double
  RMS1 : dspstat3/RMS  run=on  reset_popup=None  directionMode=Each column  dimension=1
  RMS2 : dspstat3/RMS  run=on  reset_popup=None  directionMode=Each column  dimension=1
  ROM : xbsIndex_r4/ROM  depth=16384  initVector=AGC_Gain  distributed_mem=Block RAM  rst=off  init_reg=0  en=off  latency=1  gui_display_data_type=Fixed-point  arith_type="Signed  (2's comp)"  n_bits=18  bin_pt=17  preci_type=Single  exp_width=8  frac_width=24  optimize=Area  use_rpm=on  dbl_ovrd=off  block_type=sprom
  Random Integer Generator1 : commrandsrc3/Random Integer Generator  SetSize=4  SeedSource=Auto  Seed=0  SampleTime=1/Br  SamplesPerFrame=1  OutputDataType=double  SimulateUsing=Code generation
  Rate Transition1 : RateTransition  OutPortSampleTime=Ts
  ReImPower : Subsystem
  Real Error Rate Calculation : commsink2/Error Rate Calculation  N=0  st_delay=100  cp_mode=Entire frame  subframe=[]  PMode=Port  WsName=BER  RsMode2=on  stop=off  numErr=maxNumErrs  maxBits=maxNumBits
  Real Error Rate Calculation1 : commsink2/Error Rate Calculation  N=0  st_delay=100  cp_mode=Entire frame  subframe=[]  PMode=Port  WsName=BER  RsMode2=on  stop=off  numErr=maxNumErrs  maxBits=maxNumBits
  Real-Imag to Complex : RealImagToComplex  Commented=on
  Real-Imag to Complex3 : RealImagToComplex
  Real-Imag to Complex4 : RealImagToComplex
  Real1Msb : xbsIndex_r4/Slice  nbits=1  boolean_output=on  mode=Upper Bit Location + Width  bit1=0  base1=MSB of Input  bit0=0  base0=LSB of Input  dbl_ovrd=off  block_type=slice
  Real2Msb : xbsIndex_r4/Slice  nbits=1  boolean_output=on  mode=Upper Bit Location + Width  bit1=0  base1=MSB of Input  bit0=0  base0=LSB of Input  dbl_ovrd=off  block_type=slice
  RealLock : xbsIndex_r4/Gateway Out  inherit_from_input=off  hdl_port=on  rows=1  columns=1  UseAsDAC=off  DACChannel='1'  interface=None  automatic_assignment=on  address_offset=hex2dec('00')  intf_name=''  intf_description=''  timing_constraint=None  locs_specified=off  LOCs={}  io_standard={}  block_type=gatewayout
  RealOut : xbsIndex_r4/Gateway Out  inherit_from_input=off  hdl_port=on  rows=1  columns=1  UseAsDAC=off  DACChannel='1'  interface=None  automatic_assignment=on  address_offset=hex2dec('00')  intf_name=''  intf_description=''  timing_constraint=None  locs_specified=off  LOCs={}  io_standard={}  block_type=gatewayout
  RealXord : xbsIndex_r4/Gateway Out  inherit_from_input=off  hdl_port=on  rows=1  columns=1  UseAsDAC=off  DACChannel='1'  interface=None  automatic_assignment=on  address_offset=hex2dec('00')  intf_name=''  intf_description=''  timing_constraint=None  locs_specified=off  LOCs={}  io_standard={}  block_type=gatewayout
  Relational : xbsIndex_r4/Relational  mode=a>=b  op_type=Bool  en=off  latency=0  dbl_ovrd=off  block_type=relational
  Relational1 : xbsIndex_r4/Relational  mode=a>=b  op_type=Bool  en=off  latency=0  dbl_ovrd=off  block_type=relational
  Reset : xbsIndex_r4/Gateway In  gui_display_data_type=Boolean  arith_type=Boolean  n_bits=3  bin_pt=0  preci_type=Single  exp_width=8  frac_width=24  rows=1  columns=1  quantization="Round  (unbiased: +/- Inf)"  overflow=Saturate  period=Ts  UseAsADC=off  ADCChannel='1'  interface=None  automatic_assignment=on  address_offset=hex2dec('00')  intf_name=''  intf_description=''  default_value=0  timing_constraint=None  locs_specified=off  LOCs={}  io_standard={}  inherit_from_input=off  hdl_port=on  dbl_ovrd=off  block_type=gatewayin
  Scale0 : Gain  Gain=1/4.4
  Scale1 : Gain  Gain=1/4.4
  Scope : Scope  NumInputPorts=4
  Scope1 : Scope  NumInputPorts=4
  Scope10 : Scope  NumInputPorts=2
  Scope4 : Scope  NumInputPorts=2
  Scope6 : Scope  NumInputPorts=4
  Scope7 : Scope  Commented=on
  Scope8 : Scope  NumInputPorts=8
  Scope9 : Scope  NumInputPorts=2
  Sign{,1..3} (4 alike) : Signum
  Sign3dB : xbsIndex_r4/Slice  nbits=1  boolean_output=on  mode=Upper Bit Location + Width  bit1=0  base1=MSB of Input  bit0=0  base0=LSB of Input  dbl_ovrd=off  block_type=slice
  Slice : xbsIndex_r4/Slice  nbits=14  boolean_output=off  mode=Upper Bit Location + Width  bit1=0  base1=MSB of Input  bit0=0  base0=LSB of Input  dbl_ovrd=off  block_type=slice
  Spectrum Analyzer : SpectrumAnalyzer  Commented=on
  Spectrum Analyzer2 : SpectrumAnalyzer  Commented=on
  Spectrum Analyzer3 : SpectrumAnalyzer  Commented=on
  Step : Step  Time=.0002  Before=1  After=0  SampleTime=1/Br
  Sum : Sum  Inputs=|++
  SweepLmt : xbsIndex_r4/Gateway In  gui_display_data_type=Fixed-point  arith_type=Unsigned  n_bits=11+Bits  bin_pt=0  preci_type=Single  exp_width=8  frac_width=24  rows=1  columns=1  quantization="Round  (unbiased: +/- Inf)"  overflow=Saturate  period=Ts  UseAsADC=off  ADCChannel='1'  interface=None  automatic_assignment=on  address_offset=hex2dec('00')  intf_name='axi4'  intf_description='Lead Coefficient'  default_value=5*Ts  timing_constraint=None  locs_specified=off  LOCs={}  io_standard={}  inherit_from_input=off  hdl_port=on  dbl_ovrd=off  block_type=gatewayin
  SwpRate : xbsIndex_r4/Gateway In  gui_display_data_type=Fixed-point  arith_type="Signed  (2's comp)"  n_bits=18  bin_pt=9  preci_type=Single  exp_width=8  frac_width=24  rows=1  columns=1  quantization="Round  (unbiased: +/- Inf)"  overflow=Wrap  period=Ts  UseAsADC=off  ADCChannel='1'  interface=None  automatic_assignment=on  address_offset=hex2dec('00')  intf_name='axi4'  intf_description='Lead Coefficient'  default_value=5*Ts  timing_constraint=None  locs_specified=off  LOCs={}  io_standard={}  inherit_from_input=off  hdl_port=on  dbl_ovrd=off  block_type=gatewayin
  Terminator : Terminator  Commented=on
  Terminator{1,3..8} (7 alike) : Terminator
  dB_Offset : xbsIndex_r4/Constant  const=0.5  gui_display_data_type=Fixed-point  arith_type=Signed (2's comp)  n_bits=18  bin_pt=17  preci_type=Single  exp_width=8  frac_width=24  explicit_period=on  period=Ts  equ=P=C  opselect=C  inp2=PCIN>>17  opr=+  inp1=P  carry=CIN  dbl_ovrd=off  block_type=constant
  dB_Range : xbsIndex_r4/Gateway In  gui_display_data_type=Fixed-point  arith_type=Unsigned  n_bits=16  bin_pt=10  preci_type=Single  exp_width=8  frac_width=24  rows=1  columns=1  quantization="Round  (unbiased: +/- Inf)"  overflow=Flag as error  period=Ts  UseAsADC=off  ADCChannel='1'  interface=None  automatic_assignment=on  address_offset=hex2dec('00')  intf_name=''  intf_description=''  default_value=0  timing_constraint=None  locs_specified=off  LOCs={}  io_standard={}  inherit_from_input=off  hdl_port=on  dbl_ovrd=off  block_type=gatewayin
  dB_Ratio : xbsIndex_r4/Gateway In  gui_display_data_type=Fixed-point  arith_type=Unsigned  n_bits=16  bin_pt=6  preci_type=Single  exp_width=8  frac_width=24  rows=1  columns=1  quantization="Round  (unbiased: +/- Inf)"  overflow=Flag as error  period=Ts  UseAsADC=off  ADCChannel='1'  interface=None  automatic_assignment=on  address_offset=hex2dec('00')  intf_name=''  intf_description=''  default_value=0  timing_constraint=None  locs_specified=off  LOCs={}  io_standard={}  inherit_from_input=off  hdl_port=on  dbl_ovrd=off  block_type=gatewayin
  tag scope: RawData=global, Reset_n=global, RstStep=global
  wires:
  Real-Imag to Complex/1 -> IntOffset Mixer/2
  PhaseDetect/1 -> Complex to Magnitude-Angle/1
  Conjugate/1(Out1) -> PhaseDetect/2
  NCO1/2 -> Real-Imag to Complex/1
  NCO1/1 -> Real-Imag to Complex/2
  Discrete-Time Integrator/1 -> Delay3/1, Add/1
  Gain1/1 -> Add/2
  IntOffset Mixer/1 -> AD9957-2/1(In1), Delay5/1, Conjugate/1(In1)
  Complex to Magnitude-Angle/2 -> Delay6/1, Gain1/1, Discrete-Time Integrator/1
  Complex to Real-Imag/1 -> Scope1/1, Ch0Real/1
  Complex to Real-Imag/2 -> Ch0Imag/1, Scope1/2
  Complex to Real-Imag1/2 -> Scope1/4, Ch1Imag/1
  Complex to Real-Imag1/1 -> Scope1/3, Ch1Real/1
  Int Offset Mixer/2 -> Convert/1
  Int Offset Mixer/1 -> Phase_Detect/4, Phase_Detect/1
  Conju gate/1 -> Phase_Detect/5
  Complex to Magnitude-Angle/1 -> Terminator/1
  One/1 -> Int Offset Mixer/1, Int Offset Mixer/4
  Mult/1 -> AddSub/2
  Phase Detect/1 -> Mux2/2
  Int Offset Mixer/3 -> Convert1/1
  Lead Coef/1 -> Mult/2
  Lag Coef/1 -> LimitedAccum/5(LagCoef)
  Data Type Conversion/1 -> NCO1/1
  Bipolar NCO/1(sin) -> Int Offset Mixer/5
  Bipolar NCO/2(cos) -> Int Offset Mixer/6
  Phase_Detect/1 -> Terminator1/1
  MaxRealOut/1 -> Mux5/1
  MaxImagOut/1 -> Mux6/1
  MinImagOut/1 -> Mux6/2
  MinRealOut/1 -> Mux5/2
  Convert/1 -> PhaseSlide/5(ImagSlave), Conju gate/1
  Convert1/1 -> Phase_Detect/6, PhaseSlide/6(RealSlave)
  Mux5/1 -> LocksAndMinMax/3
  Mux6/1 -> LocksAndMinMax/4
  Bias1/1 -> Scale1/1  "AgcCh1"
  Bias/1 -> Scale0/1  "AgcCh0"
  Mult2/1 -> ReImPower/3(Real2), AddReals/1
  Mult4/1 -> ReImPower/5(Real3), AddReals/2
  Mult5/1 -> ReImPower/6(Imag3), AddImags/2
  Mult3/1 -> ReImPower/4(Imag2), AddImags/1
  AddReals/1 -> ReImPower/1(Real1), RealOut/1
  ImagOut/1 -> Integrate and Dump2/1, Scope/4
  AddImags/1 -> ReImPower/2(Imag1), ImagOut/1
  Constant11/1 -> Lag Coef/1
  Constant12/1 -> Lead Coef/1
  AWGN Channel1/1 -> Gain5/1
  Gain5/1 -> Lowpass Filter1/1
  Phase_Detect/2 -> Cordic ATan/1(Imag)
  Phase_Detect/3 -> Cordic ATan/2(Real)
  ExtOffset Mixer1/1 -> AWGN Channel2/1
  Complex to Real-Imag5/1 -> Mux1/1
  Complex to Real-Imag5/2 -> Mux1/2
  Lag Out/1 -> Scope8/7, Mux3/2  "LagOut"
  Delay3/1 -> Mux3/1
  Delay5/1 -> Complex to Real-Imag5/1
  Delay6/1 -> Mux2/1
  AD9957-2/1(Out1) -> Spectrum Analyzer2/1
  Real1Msb/1 -> Logical/1
  Real2Msb/1 -> Logical/2
  RealXord/1 -> Mux9/1
  Imag1Msb/1 -> Logical1/1
  Imag2Msb/1 -> Logical1/2
  ImagXord/1 -> Mux9/2
  RealLock/1 -> Mux10/2, Display/1
  Mux9/1 -> LocksAndMinMax/2
  Logical1/1 -> LockImag/2(Sub), Mux7/1, ImagXord/1
  LockImag/1(Out) -> Relational1/1, ImagLock/1
  Mux7/1 -> LockImag/1(In)
  ImagLock/1 -> Display4/1, Mux10/1
  Mux10/1 -> [Locks], LocksAndMinMax/1  "LockDetectors"
  Delay/1 -> Data Type Conversion/1
  Mux3/1 -> Loop Filter Scope/3  "LagOut"
  Mux4/1 -> Loop Filter Scope/4  "NCO Controls"
  Delay4/1 -> Mux4/1
  NCO Control Out/1 -> Mux4/2
  Ch0Imag/1 -> ChanSwapper/2(Ch1Imag)
  Ch1Real/1 -> ChanSwapper/3(Ch2Real)
  Ch1Imag/1 -> ChanSwapper/4(Ch2Imag)
  Ch0Real/1 -> ChanSwapper/1(Ch1Real)
  ChanSwapper/4(MinImag) -> Int Offset Mixer/2
  ChanSwapper/3("MinReal ") -> Int Offset Mixer/3
  Constant4/1 -> Mux7/2
  Constant5/1 -> Mux7/3
  Logical/1 -> LockReal/2(Sub), Mux8/1, RealXord/1
  Constant6/1 -> Mux8/2
  Constant9/1 -> Mux8/3
  Negate1/1 -> NCO Control Out/1, Bipolar NCO/2(Inc)
  ChanSwapper/5(Ch1SelDly) -> Delay11/1, Inverter4/1
  AddSub/1 -> Negate1/1
  Cordic ATan/1(Phase) -> Negater2/2(In)
  Delay10/1 -> Delay12/1
  Add/1 -> Delay4/1, Delay/1
  Relational1/1 -> Logical2/2
  Relational/1 -> Logical2/1
  Locked/1 -> Display7/1
  Mux2/1 -> Loop Filter Scope/2  "PhaseErrs"
  LimitedAccum/1(Out) -> AddSub/1, Lag Out/1
  Negater2/1(Out) -> Mult/1, LimitedAccum/2(PhaseErr), Phase Detect/1
  SweepLmt/1 -> LimitedAccum/1(Limit)
  Constant13/1 -> SweepLmt/1
  ChanSwapper/1(MaxReal) -> Delay1/1
  ChanSwapper/2(MaxImag) -> Delay2/1
  Delay2/1 -> PhaseSlide/3(ImagMaster), Phase_Detect/2
  Delay1/1 -> PhaseSlide/2(RealMaster), Phase_Detect/3
  Constant14/1 -> SwpRate/1
  SwpRate/1 -> LimitedAccum/4(SwpRate)
  [Locked] -> LimitedAccum/3(Locked)
  Delay7/1 -> Complex to Real-Imag2/1
  Product1/1 -> Mux11/2
  Product/1 -> Mux11/1
  Mux/1 -> BERs/1
  Mux13/1 -> BERs/2
  Integrate and Dump1/1 -> Product/2, Mux/2, Sign/1
  GainOutMax/1 -> Scope9/2, Display9/1
  [RawData] -> Gain3/1
  Real Error Rate Calculation/1 -> Display16/1, Demux/1
  Complex to Real-Imag2/1 -> Integrate and Dump1/1, Scope/2
  Integrate and Dump2/1 -> Product1/1, Sign3/1, Mux13/1
  Integrate and Dump3/1 -> Product1/2, Sign2/1, Mux13/2
  Complex to Real-Imag2/2 -> Integrate and Dump3/1, Scope/3
  RealOut/1 -> Integrate and Dump4/1, Scope/1
  Sign/1 -> Real Error Rate Calculation/1
  Sign1/1 -> Real Error Rate Calculation/2
  [Ch0GtCh1] -> ChanSwapper/5(Ch1Sel)
  Inverter1/1 -> Int Offset Mixer/7, [Reset_n]
  [Reset_n] -> Phase_Detect/7
  [Reset_n] -> LockImag/3(Rst_n), LockReal/3(Rst_n)
  Gain 20dB/V1/1 -> Bias1/1
  GainOutMax3/1 -> Gain4/1
  ReImPower/1(Power1) -> GainOutMax3/1
  AGC Ch1/1 -> RMS1/1, BER/1(In), Spectrum Analyzer/1, IntOffset Mixer/1, Delay9/1  "Ch1"
  Gain4/1 -> Scope6/1, Display1/1  "Sum"
  GainOutMax2/1 -> Gain7/1
  Gain7/1 -> Scope6/2, Display2/1  "Master"
  GainOutMax1/1 -> Gain8/1
  Gain8/1 -> Scope6/3, Display6/1  "Slave"
  ReImPower/3(Power3) -> GainOutMax1/1
  ReImPower/2(Power2) -> GainOutMax2/1
  Manual Switch5/1 -> AWGN Channel1/1, ExtOffset Mixer1/1, [RawData]
  Constant21/1 -> Reset/1
  Gain3/1 -> Delay7/1
  AddressSlice/1 -> Display8/1
  BER/1(Out1) -> Mux14/1
  AGC Ch2/1 -> BER1/1(In), RMS2/1, PhaseDetect/1, Spectrum Analyzer3/1, Complex to Real-Imag1/1  "Ch2"
  BER1/1(Out1) -> Mux14/2
  Mux16/1 -> Display11/1
  Mux14/1 -> Display14/1
  Mux15/1 -> Display13/1
  Lowpass Filter1/1 -> AGC Ch1/1  "Ch1"
  RMS2/1 -> Mux15/2
  RMS1/1 -> Mux15/1
  Manual Reset/1 -> Real Error Rate Calculation/3, Real Error Rate Calculation1/3, [RstStep]
  Mux11/1 -> BERs/3
  AWGN Channel2/1 -> Gain6/1
  Gain6/1 -> Lowpass Filter2/1
  Lowpass Filter2/1 -> AGC Ch2/1  "Ch1"
  [RstStep] -> Display15/1
  Mux19/1 -> GainOutMax/1, Mult3/2, Mult2/2
  Sign2/1 -> Real Error Rate Calculation1/1
  Sign3/1 -> Real Error Rate Calculation1/2
  Real Error Rate Calculation1/1 -> Demux1/1, Display17/1
  Demux1/1 -> Mux16/2
  Demux/1 -> Mux16/1
  Address1/1 -> Display18/1
  Manual Switch1/1 -> Gain 20dB/V/1, AGCtoAWGN1/1(AGC)
  Gain 20dB/V/1 -> Bias/1
  AGCtoAWGN1/1(Variance) -> AWGN Channel1/2
  AGCtoAWGN2/1(Variance) -> AWGN Channel2/2
  Reset/1 -> [Reset], Inverter1/1, Bipolar NCO/1(Rst)
  AddSub1/1 -> NeverZero/2, Delay13/1, AllZeros/1, AllOnes/1  "GainSlave"
  Constant3/1 -> OneMinusSlave/1
  LockReal1/1 -> LockThresh/1, Relational1/2, Relational/2
  Constant10/1 -> LockThreshold/1
  Constant15/1 -> LockHysterisis/1
  LockThreshold/1 -> LockReal1/1
  LockHysterisis/1 -> LockReal1/2
  Logical2/1 -> LockReal1/3, Locked/1, [Locked]
  LockThresh/1 -> Display19/1
  Delay9/1 -> Complex to Real-Imag/1
  Demux/2 -> Terminator3/1
  Demux/3 -> Terminator4/1
  Demux1/2 -> Terminator5/1
  Demux1/3 -> Terminator6/1
  LockReal/1(Out) -> RealLock/1, Relational/1
  Mux8/1 -> LockReal/1(In)
  IIR_Out1/1 -> Scope8/2  "SlaveGain"
  GainOutMin/1 -> Scope9/1, Display10/1  "Diff"
  IIR_Out5/1 -> Scope8/4  "X8Filtered"
  IIR_Out4/1 -> Scope8/3  "0Gt1"
  [Locks] -> Scope8/6  "Locks"
  IIR_Out2/1 -> Scope8/5  "Locked"
  Mult6/1 -> IIR_Out4/1, AddSub1/1
  Ch0AGC/1 -> IIR_Out6/1, DiffDB/1
  Ch1AGC/1 -> IIR_Out7/1, DiffDB/2
  Constant23/1 -> Manual Switch6/1
  Constant24/1 -> Manual Switch6/2
  Manual Switch6/1 -> Ch0GtCh1/1
  Constant26/1 -> Manual Switch4/1
  Constant25/1 -> Manual Switch4/2
  Manual Switch4/1 -> OverrideCh/1
  OverrideCh/1 -> Mux18/1
  Ch0GtCh1/1 -> Mux20/1
  Scale0/1 -> Ch0AGC/1
  Sum/1 -> Ch1AGC/1
  Scale1/1 -> Sum/1
  Constant17/1 -> Sum/2
  dB_Ratio/1 -> Mult1/1
  Divide/1 -> dB_Ratio/1
  High/1 -> Mux20/2
  High1/1 -> Mux20/3
  Mux20/1 -> Mux18/3
  DiffDB/1 -> Mux18/2
  Constant20/1 -> Divide/1
  [dB_Range] -> Divide/2
  Mult1/1 -> Slice/1, Address1/1, IIR_Out5/1, Current±3dB/1, IIR_Out/1
  Sign3dB/1 -> Delay8/1
  1.5dBHysteresis/1 -> Current±3dB/2
  Delay8/1 -> Inverter3/1, Current±3dB/3
  Inverter3/1 -> [Ch0GtCh1], Inverter5/1, AGC0_GT_AGC1/1
  Logical4/1 -> Delay8/3
  AGC0_GT_AGC1/1 -> Scope8/1, Display3/1  "Agc0GtAgc1"
  Current±3dB/1 -> Sign3dB/1
  Inverter2/1 -> Logical4/1
  [Locked] -> Inverter2/1
  AllOnes/1 -> Logical5/1
  AllZeros/1 -> NeverZero/1, Logical5/2
  [Reset] -> Delay8/2
  Constant22/1 -> [dB_Range], dB_Range/1
  Mux17/1 -> Scope8/8, BERs/4, Scope6/4  "Gains"
  AGC0/1 -> Manual Switch1/1
  AGC1/1 -> Manual Switch3/1
  Manual Switch3/1 -> Gain 20dB/V1/1, AGCtoAWGN2/1(AGC)
  [Reset] -> LimitedAccum/6(Rst)
  Logical5/1 -> Logical4/2, IIR_Out2/1
  Fade1/1 -> Manual Switch3/2, Mux17/2
  Fade0/1 -> Mux17/1, Manual Switch1/2
  IIR_Out/1 -> Scope4/1
  Mux18/1 -> IIR_Out3/1, Mult1/2
  IIR_Out3/1 -> Scope4/2
  IIR_Out7/1 -> Scope10/2
  IIR_Out6/1 -> Scope10/1
  Slice/1 -> AddressSlice/1, ROM/1
  ROM/1 -> Mult6/2
  dB_Offset/1 -> AddSub1/2
  dB_Range/1 -> Mult6/1
  Inverter4/1 -> Bipolar NCO/3(Conj)
  NCO HDL Optimized1/1 -> Real-Imag to Complex3/2
  NCO HDL Optimized1/2 -> Real-Imag to Complex3/1
  Real-Imag to Complex3/1 -> ExtOffset Mixer1/2, Scope7/1
  Random Integer Generator1/1 -> Rate Transition1/1
  Rate Transition1/1 -> QPSK Modulator Baseband1/1
  Constant1/1 -> NCO HDL Optimized1/1
  NCO HDL Optimized1/3 -> Terminator8/1
  CW/1 -> Real-Imag to Complex4/2
  CW/2 -> Real-Imag to Complex4/1
  Constant2/1 -> CW/1
  CW/3 -> Terminator7/1
  QPSK Modulator Baseband1/1 -> Manual Switch5/1
  Real-Imag to Complex4/1 -> Manual Switch5/2
  Bipolar NCO/3(phase) -> [Phase]
  Mux1/1 -> Loop Filter Scope/1
  [Phase] -> PhaseSlide/4(PhaseIn)
  PhaseSlide/3(RealSlaveOut) -> Real2Msb/1, MinRealOut/1, Mult4/1
  PhaseSlide/4(ImagSlaveOut) -> Imag2Msb/1, MinImagOut/1, Mult5/1
  PhaseSlide/2(ImagMasterOut) -> Imag1Msb/1, Mult3/1, MaxImagOut/1
  PhaseSlide/1(RealMasterOut) -> Mult2/1, MaxRealOut/1, Real1Msb/1
  Delay11/1 -> Delay10/1
  Delay12/1 -> PhaseSlide/1(ChSel), Negater2/1(Neg)
  Integrate and Dump4/1 -> Sign1/1, Mux/1, Product/1
  Step/1 -> Manual Reset/1
  Constant/1 -> Manual Reset/2
  Mux12/1 -> GainOutMin/1, Mult5/2, Mult4/2
  OneMinusSlave/1 -> Mux12/3, Mux19/2
  Inverter5/1 -> Mux12/1, Mux19/1
  NeverZero/1 -> Mux19/3, Mux12/2, IIR_Out1/1, OneMinusSlave/2
  Delay13/1 -> NeverZero/3
